simulink model "Dyn_6DoF_v2_0_R2015B"  (R2015b)
settings: Solver=ode4  SolverMode=SingleTasking  StartTime=0.0  StopTime=simInit.TSIM  FixedStep=simInit.dt  MaxStep=simInit.dt  RelTol=1e-3
InitFcn:
  | close all
undefined symbols (not defined in the file): act, base_windspeed, constr, DE2019, DiscIntNeverNeededParam, ENVMT, Lbooth, loiterStates, omega_rate_max, params, simInit, T, winchParameter
libraries: simulink x41, simulink_extras x4, dspsigops x1
(part 2 of 6)

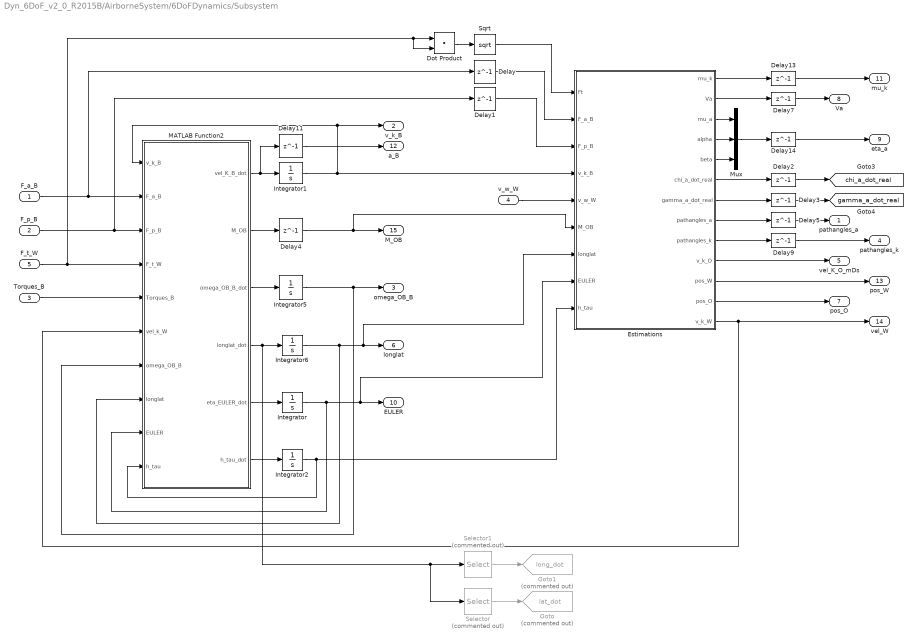
== system Dyn_6DoF_v2_0_R2015B/AirborneSystem/6DoFDynamics/Subsystem ==
  F_a_B : Inport  PortDimensions=[3,1]
  F_p_B : Inport  Port=2
  Torques_B : Inport  Port=3  PortDimensions=[3,1]
  v_w_W : Inport  Port=4  PortDimensions=[3,1]
  F_t_W : Inport  Port=5
  Delay{,1,11,14} (4 alike) : Delay  DelayLength=1  InitialCondition=zeros(3,1)
  Delay13 : Delay  DelayLength=1  InitialCondition=0
  Delay2 : Delay  DelayLength=1
  Delay3 : Delay  DelayLength=1
  Delay4 : Delay  DelayLength=1  InitialCondition=eye(3)
  Delay5 : Delay  DelayLength=1  InitialCondition=zeros(2,1)
  Delay7 : Delay  DelayLength=1  InitialCondition=simInit.vel_B_init(1)
  Delay9 : Delay  DelayLength=1  InitialCondition=zeros(2,1)
  Dot Product : DotProduct  InputSameDT=on  OutDataTypeStr=Inherit: Inherit via internal rule
  Estimations : MATLAB Function  TreatAsAtomicUnit=on
  Goto : Goto  Commented=on  GotoTag=lat_dot  TagVisibility=global
  Goto1 : Goto  Commented=on  GotoTag=long_dot  TagVisibility=global
  Integrator : Integrator  InitialCondition=simInit.eta_init  WrapState=on
  Integrator1 : Integrator  InitialCondition=simInit.vel_B_init
  Integrator2 : Integrator  InitialCondition=norm(simInit.pos_O_init)
  Integrator5 : Integrator  InitialCondition=zeros(3,1)
  Integrator6 : Integrator  InitialCondition=[simInit.long_init;simInit.lat_init]  WrapState=on
  MATLAB Function2 : MATLAB Function  TreatAsAtomicUnit=on
  Mux : Mux  Inputs=3
  Selector : Selector  Commented=on  InputPortWidth=2  IndexOptions=Index vector (dialog)  Indices=2  OutputSizes=1
  Selector1 : Selector  Commented=on  InputPortWidth=2  IndexOptions=Index vector (dialog)  Indices=1  OutputSizes=1
  Sqrt : Sqrt  SaturateOnIntegerOverflow=on
  pathangles_a : Outport  PortDimensions=[2,1]
  v_k_B : Outport  Port=2  PortDimensions=[3,1]
  omega_OB_B : Outport  Port=3  PortDimensions=[3,1]
  pathangles_k : Outport  Port=4  PortDimensions=[2,1]
  vel_K_O_mDs : Outport  Port=5  PortDimensions=[3,1]
  longlat : Outport  Port=6  PortDimensions=[2,1]
  pos_O : Outport  Port=7  PortDimensions=[3,1]
  Va : Outport  Port=8  PortDimensions=1
  eta_a : Outport  Port=9  PortDimensions=[3,1]
  EULER : Outport  Port=10  PortDimensions=[3,1]
  mu_k : Outport  Port=11  PortDimensions=1
  a_B : Outport  Port=12  PortDimensions=[3,1]
  pos_W : Outport  Port=13  PortDimensions=[3,1]
  vel_W : Outport  Port=14  PortDimensions=[3,1]
  M_OB : Outport  Port=15  PortDimensions=[3,3]
  tag scope: chi_a_dot_real=global, gamma_a_dot_real=global
  wires:
  Delay5/1 -> pathangles_a/1
  Delay4/1 -> M_OB/1, Estimations/6(M_OB)
  Torques_B/1 -> MATLAB Function2/5(Torques_B)
  MATLAB Function2/2(M_OB) -> Delay4/1
  F_a_B/1 -> MATLAB Function2/2(F_a_B), Delay/1
  Mux/1 -> Delay14/1
  MATLAB Function2/3(omega_OB_B_dot) -> Integrator5/1
  MATLAB Function2/4(longlat_dot) -> Integrator6/1, Selector/1, Selector1/1
  MATLAB Function2/1(vel_K_B_dot) -> Delay11/1, Integrator1/1
  v_w_W/1 -> Estimations/5(v_w_W)
  Integrator1/1 -> Estimations/4(v_k_B), MATLAB Function2/1(v_k_B), v_k_B/1
  F_p_B/1 -> MATLAB Function2/3(F_p_B), Delay1/1
  Estimations/8(pathangles_a) -> Delay5/1
  Estimations/9(pathangles_k) -> Delay9/1
  Estimations/2(Va) -> Delay7/1
  Delay7/1 -> Va/1
  Estimations/3(mu_a) -> Mux/1
  Delay2/1 -> [chi_a_dot_real]
  Estimations/6(chi_a_dot_real) -> Delay2/1
  Estimations/7(gamma_a_dot_real) -> Delay3/1
  Delay3/1 -> [gamma_a_dot_real]
  MATLAB Function2/5(eta_EULER_dot) -> Integrator/1
  Integrator/1 -> MATLAB Function2/9(EULER), Estimations/8(EULER), EULER/1
  Integrator5/1 -> MATLAB Function2/7(omega_OB_B), omega_OB_B/1
  Estimations/1(mu_k) -> Delay13/1
  Integrator6/1 -> MATLAB Function2/8(longlat), Estimations/7(longlat), longlat/1
  Delay13/1 -> mu_k/1
  Delay14/1 -> eta_a/1
  Delay9/1 -> pathangles_k/1
  Estimations/4(alpha) -> Mux/2
  Estimations/5(beta) -> Mux/3
  F_t_W/1 -> MATLAB Function2/4(F_t_W), Dot Product/1, Dot Product/2
  Dot Product/1 -> Sqrt/1
  Delay11/1 -> a_B/1
  MATLAB Function2/6(h_tau_dot) -> Integrator2/1
  Integrator2/1 -> MATLAB Function2/10(h_tau), Estimations/9(h_tau)
  Estimations/12(pos_O) -> pos_O/1
  Estimations/13(v_k_W) -> MATLAB Function2/6(vel_k_W), vel_W/1
  Estimations/11(pos_W) -> pos_W/1
  Estimations/10(v_k_O) -> vel_K_O_mDs/1
  Delay/1 -> Estimations/2(F_a_B)
  Delay1/1 -> Estimations/3(F_p_B)
  Sqrt/1 -> Estimations/1(Ft)
  Selector/1 -> Goto/1
  Selector1/1 -> Goto1/1

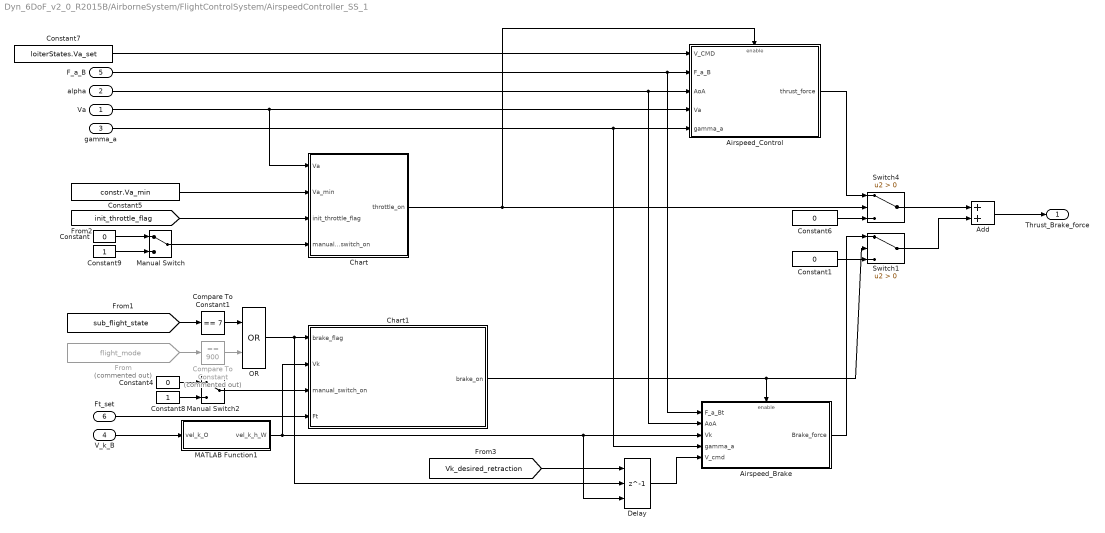
== system Dyn_6DoF_v2_0_R2015B/AirborneSystem/FlightControlSystem/AirspeedController_SS_1 ==
  Va : Inport
  alpha : Inport  Port=2
  gamma_a : Inport  Port=3
  V_k_B : Inport  Port=4
  F_a_B : Inport  Port=5
  Ft_set : Inport  Port=6
  Add : Sum
  Airspeed_Brake : Subsystem
  Airspeed_Control : Subsystem
  Chart : Stateflow chart  TreatAsAtomicUnit=on
  Chart1 : Stateflow chart  TreatAsAtomicUnit=on  mask{Ft_retract=params.F_t_retraction_set*params.F_t_traction_set, Vk_min=30}
      mask prompts: Ft_retract "Retraction force"; Vk_min "Minimum Vk"
  Compare To Constant : simulink/Logic and Bit Operations/Compare To Constant  Commented=on  relop===  const=900  OutDataTypeStr=boolean
  Compare To Constant1 : simulink/Logic and Bit Operations/Compare To Constant  relop===  const=7  OutDataTypeStr=boolean
  Constant{,1,4,6} (4 alike) : Constant  Value=0
  Constant5 : Constant  Value=constr.Va_min
  Constant7 : Constant  Value=loiterStates.Va_set
  Constant8 : Constant
  Constant9 : Constant
  Delay : Delay  DelayLength=1  InitialConditionSource=Input port  ExternalReset=Rising
      settings: InputPortMap=u0,r5,p4
  From : From  Commented=on  GotoTag=flight_mode  TagVisibility=global
  MATLAB Function1 : MATLAB Function  TreatAsAtomicUnit=on
  Manual Switch : ManualSwitch
  Manual Switch2 : ManualSwitch
  OR : Logic  Operator=OR  IconShape=distinctive  AllPortsSameDT=off  OutDataTypeStr=boolean
  Switch1 : Switch  Criteria=u2 > Threshold
  Switch4 : Switch  Criteria=u2 > Threshold
  Thrust_Brake_force : Outport
  wires:
  Switch1/1 -> Add/2
  Constant1/1 -> Switch1/3
  [Vk_desired_retraction] -> Delay/1
  Compare To Constant/1 -> OR/2
  Compare To Constant1/1 -> OR/1
  MATLAB Function1/1(vel_k_h_W) -> Chart1/2(Vk), Delay/3, Airspeed_Brake/3(Vk)
  V_k_B/1 -> MATLAB Function1/1(vel_k_O)
  Delay/1 -> Airspeed_Brake/5(V_cmd)
  Constant8/1 -> Manual Switch2/2
  Constant4/1 -> Manual Switch2/1
  Add/1 -> Thrust_Brake_force/1
  From/1 -> Compare To Constant/1
  [sub_flight_state] -> Compare To Constant1/1
  OR/1 -> Chart1/1(brake_flag), Delay/2
  Manual Switch2/1 -> Chart1/3(manual_switch_on)
  Ft_set/1 -> Chart1/4(Ft)
  Airspeed_Brake/1(Brake_force) -> Switch1/1
  Chart1/1(brake_on) -> Switch1/2, Airspeed_Brake/Enable
  Airspeed_Control/1(thrust_force) -> Switch4/1
  Constant5/1 -> Chart/2(Va_min)
  Va/1 -> Chart/1(Va), Airspeed_Control/4(Va)
  Chart/1(throttle_on) -> Switch4/2, Airspeed_Control/Enable
  Constant9/1 -> Manual Switch/2
  [init_throttle_flag] -> Chart/3(init_throttle_flag)
  alpha/1 -> Airspeed_Control/3(AoA), Airspeed_Brake/2(AoA)
  Constant7/1 -> Airspeed_Control/1(V_CMD)
  Manual Switch/1 -> Chart/4(manual_switch_on)
  Constant/1 -> Manual Switch/1
  Constant6/1 -> Switch4/3
  F_a_B/1 -> Airspeed_Control/2(F_a_B), Airspeed_Brake/1(F_a_Bt)
  gamma_a/1 -> Airspeed_Control/5(gamma_a), Airspeed_Brake/4(gamma_a)
  Switch4/1 -> Add/1

== system Dyn_6DoF_v2_0_R2015B/AirborneSystem/FlightControlSystem/AttitudeAndRateLoop ==
  mu_a_cmd : Inport
  M_a_B_est : Inport  Port=2
  flightMode : Inport  Port=3
  alpha_a_cmd : Inport  Port=4
  StateEstimation_Bus : Inport  Port=5
  AttitudeController : Subsystem
  Compare To Constant : simulink/Logic and Bit Operations/Compare To Constant  relop===  const=6  OutDataTypeStr=boolean
  RateLoop : Subsystem
  u_rb : Outport
  wires:
  M_a_B_est/1 -> RateLoop/3(M_a_B_est)
  RateLoop/1(u_rb) -> u_rb/1
  mu_a_cmd/1 -> AttitudeController/2(mu_a_cmd)
  AttitudeController/1(omega_OB_B_cmd) -> RateLoop/2(omega_OB_B_cmd)
  alpha_a_cmd/1 -> AttitudeController/3(alpha_a_cmd)
  StateEstimation_Bus/1 -> RateLoop/1(StateEstimation_Bus), AttitudeController/1(StateEstimation_Bus)
  flightMode/1 -> Compare To Constant/1
  Compare To Constant/1 -> AttitudeController/4(reset)

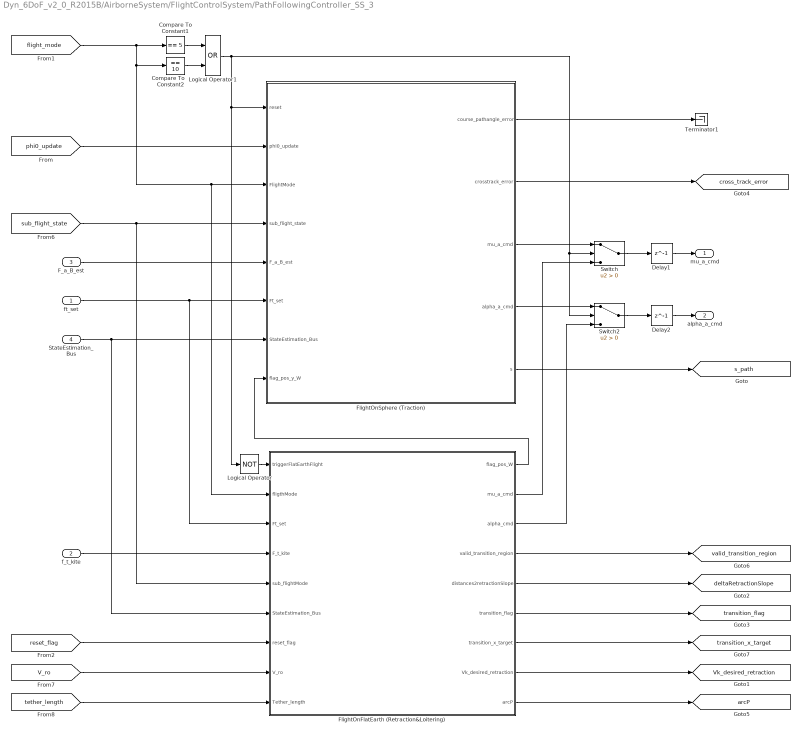
== system Dyn_6DoF_v2_0_R2015B/AirborneSystem/FlightControlSystem/PathFollowingController_SS_3 ==
  ft_set : Inport
  f_t_kite : Inport  Port=2
  F_a_B_est : Inport  Port=3  PortDimensions=[3,1]
  StateEstimation_Bus : Inport  Port=4
  Compare To Constant1 : simulink/Logic and Bit Operations/Compare To Constant  relop===  const=5  OutDataTypeStr=boolean
  Compare To Constant2 : simulink/Logic and Bit Operations/Compare To Constant  relop===  const=10  OutDataTypeStr=boolean
  Delay1 : Delay  DelayLength=1
  Delay2 : Delay  DelayLength=1
  FlightOnFlatEarth (Retraction&Loitering) : Subsystem
  FlightOnSphere (Traction) : Subsystem
  Logical Operator : Logic  Operator=NOT  AllPortsSameDT=off  OutDataTypeStr=boolean
  Logical Operator1 : Logic  Operator=OR  AllPortsSameDT=off  OutDataTypeStr=boolean
  Switch : Switch  Criteria=u2 > Threshold
  Switch2 : Switch  Criteria=u2 > Threshold
  Terminator1 : Terminator
  mu_a_cmd : Outport  PortDimensions=1
  alpha_a_cmd : Outport  Port=2  PortDimensions=1
  tag scope: Vk_desired_retraction=global, arcP=global, cross_track_error=global, deltaRetractionSlope=global, s_path=global, transition_flag=global, transition_x_target=global, valid_transition_region=global
  wires:
  FlightOnFlatEarth (Retraction&Loitering)/9(arcP) -> [arcP]
  [sub_flight_state] -> FlightOnSphere (Traction)/4(sub_flight_state), FlightOnFlatEarth (Retraction&Loitering)/5(sub_flightMode)
  [tether_length] -> FlightOnFlatEarth (Retraction&Loitering)/9(Tether_length)
  [V_ro] -> FlightOnFlatEarth (Retraction&Loitering)/8(V_ro)
  FlightOnFlatEarth (Retraction&Loitering)/8(Vk_desired_retraction) -> [Vk_desired_retraction]
  FlightOnFlatEarth (Retraction&Loitering)/7(transition_x_target) -> [transition_x_target]
  FlightOnFlatEarth (Retraction&Loitering)/1(flag_pos_W) -> FlightOnSphere (Traction)/8(flag_pos_y_W)
  FlightOnFlatEarth (Retraction&Loitering)/5(distances2retractionSlope) -> [deltaRetractionSlope]
  [reset_flag] -> FlightOnFlatEarth (Retraction&Loitering)/7(reset_flag)
  FlightOnFlatEarth (Retraction&Loitering)/6(transition_flag) -> [transition_flag]
  [phi0_update] -> FlightOnSphere (Traction)/2(phi0_update)
  FlightOnSphere (Traction)/5(s) -> [s_path]
  Compare To Constant2/1 -> Logical Operator1/2
  Compare To Constant1/1 -> Logical Operator1/1
  [flight_mode] -> Compare To Constant2/1, FlightOnSphere (Traction)/3(FlightMode), FlightOnFlatEarth (Retraction&Loitering)/2(fligthMode), Compare To Constant1/1
  FlightOnSphere (Traction)/2(crosstrack_error) -> [cross_track_error]
  FlightOnSphere (Traction)/1(course_pathangle_error) -> Terminator1/1
  FlightOnSphere (Traction)/3(mu_a_cmd) -> Switch/1
  FlightOnSphere (Traction)/4(alpha_a_cmd) -> Switch2/1
  F_a_B_est/1 -> FlightOnSphere (Traction)/5(F_a_B_est)
  f_t_kite/1 -> FlightOnFlatEarth (Retraction&Loitering)/4(F_t_kite)
  Switch2/1 -> Delay2/1
  Switch/1 -> Delay1/1
  Delay1/1 -> mu_a_cmd/1
  Delay2/1 -> alpha_a_cmd/1
  ft_set/1 -> FlightOnSphere (Traction)/6(Ft_set), FlightOnFlatEarth (Retraction&Loitering)/3(Ft_set)
  Logical Operator/1 -> FlightOnFlatEarth (Retraction&Loitering)/1(triggerFlatEarthFlight)
  FlightOnFlatEarth (Retraction&Loitering)/2(mu_a_cmd) -> Switch/3
  FlightOnFlatEarth (Retraction&Loitering)/3(alpha_cmd) -> Switch2/3
  FlightOnFlatEarth (Retraction&Loitering)/4(valid_transition_region) -> [valid_transition_region]
  Logical Operator1/1 -> Switch2/2, Switch/2, Logical Operator/1, FlightOnSphere (Traction)/1(reset)
  StateEstimation_Bus/1 -> FlightOnFlatEarth (Retraction&Loitering)/6(StateEstimation_Bus), FlightOnSphere (Traction)/7(StateEstimation_Bus)

== system Dyn_6DoF_v2_0_R2015B/AirborneSystem/ForcesAndTorques/Subsystem Reference_SS_4 ==
  u_cmd : Inport
  Aileron1 : Subsystem  mask(Rate and Position Limited Servo){freq=act.aileron.w0/(2*pi), RL=act.aileron.rl, POS_hi=act.aileron.max_deflection, POS_lo=act.aileron.min_deflection, Bias=act.aileron.bias}
      mask prompts: freq "Bandwidth, Hz"; RL "Rate Limit:"; POS_hi "Position Limit High:"; POS_lo "Position Limit Low:"; Bias "Bias Value:"
      mask help:
      | First order transfer function: w/(s+w), with rate and position limits
      | and output bias level.
      mask Display:
      | text(.48,.55,sprintf('%3.1f Hz\nBW',freq),'horizontalAlignment','center');
      | 
      | text(0.18,0.45,sprintf('|d/dt|\n<%0.1f',RL),'horizontalAlignment','center');
      | 
      | text(0.88,0.85,num2str(POS_hi),'horizontalAlignment', 'center');
      | text(0.88,0.2,num2str(POS_lo),'horizontalAlignment', 'center');
      | text(0.73,0.5,'P\nL');
      | 
      | 
      | plot([0.83 0.87 0.93 0.97],[0.4 0.4 0.6 0.6]);
      | plot([0.81 0.99],[0.5 0.5]);
      | plot([0.9 0.9],[0.3 0.7]);
      | plot([0.81 0.99 0.99 0.81 0.81],[0.3 0.3 0.7 0.7 0.3]);
  Delay1 : Delay  Commented=on  DelayLength=1  InitialCondition=0
  Delay2 : Delay  Commented=on  DelayLength=1  InitialCondition=0
  Delay3 : Delay  Commented=on  DelayLength=1  InitialCondition=0
  Delay4 : Delay  DelayLength=1  InitialCondition=0
  Delay5 : Delay  DelayLength=1  InitialCondition=0
  Delay6 : Delay  DelayLength=1  InitialCondition=0
  Demux : Demux  Outputs=3
  Elevator : Subsystem  mask(Rate and Position Limited Servo){freq=act.elevator.w0/(2*pi), RL=act.elevator.rl, POS_hi=act.elevator.max_deflection, POS_lo=act.elevator.min_deflection, Bias=act.elevator.bias}
      mask prompts: freq "Bandwidth, Hz"; RL "Rate Limit:"; POS_hi "Position Limit High:"; POS_lo "Position Limit Low:"; Bias "Bias Value:"
      mask help:
      | First order transfer function: w/(s+w), with rate and position limits
      | and output bias level.
      mask Display:
      | text(.48,.55,sprintf('%3.1f Hz\nBW',freq),'horizontalAlignment','center');
      | 
      | text(0.18,0.45,sprintf('|d/dt|\n<%0.1f',RL),'horizontalAlignment','center');
      | 
      | text(0.88,0.85,num2str(POS_hi),'horizontalAlignment', 'center');
      | text(0.88,0.2,num2str(POS_lo),'horizontalAlignment', 'center');
      | text(0.73,0.5,'P\nL');
      | 
      | 
      | plot([0.83 0.87 0.93 0.97],[0.4 0.4 0.6 0.6]);
      | plot([0.81 0.99],[0.5 0.5]);
      | plot([0.9 0.9],[0.3 0.7]);
      | plot([0.81 0.99 0.99 0.81 0.81],[0.3 0.3 0.7 0.7 0.3]);
  Manual Switch : ManualSwitch  CurrentSetting=0
  Mux1 : Mux  Inputs=3
  Mux2 : Mux  Inputs=3
  Rudder1 : Subsystem  mask(Rate and Position Limited Servo){freq=act.rudder.w0/(2*pi), RL=act.rudder.rl, POS_hi=act.rudder.max_deflection, POS_lo=act.rudder.min_deflection, Bias=act.rudder.bias}
      mask prompts: freq "Bandwidth, Hz"; RL "Rate Limit:"; POS_hi "Position Limit High:"; POS_lo "Position Limit Low:"; Bias "Bias Value:"
      mask help:
      | First order transfer function: w/(s+w), with rate and position limits
      | and output bias level.
      mask Display:
      | text(.48,.55,sprintf('%3.1f Hz\nBW',freq),'horizontalAlignment','center');
      | 
      | text(0.18,0.45,sprintf('|d/dt|\n<%0.1f',RL),'horizontalAlignment','center');
      | 
      | text(0.88,0.85,num2str(POS_hi),'horizontalAlignment', 'center');
      | text(0.88,0.2,num2str(POS_lo),'horizontalAlignment', 'center');
      | text(0.73,0.5,'P\nL');
      | 
      | 
      | plot([0.83 0.87 0.93 0.97],[0.4 0.4 0.6 0.6]);
      | plot([0.81 0.99],[0.5 0.5]);
      | plot([0.9 0.9],[0.3 0.7]);
      | plot([0.81 0.99 0.99 0.81 0.81],[0.3 0.3 0.7 0.7 0.3]);
  Saturation : Saturate  Commented=on  UpperLimit=act.aileron.max_deflection  LowerLimit=act.aileron.min_deflection
  Saturation1 : Saturate  Commented=on  UpperLimit=act.elevator.max_deflection  LowerLimit=act.elevator.min_deflection
  Saturation2 : Saturate  Commented=on  UpperLimit=act.rudder.max_deflection  LowerLimit=act.rudder.min_deflection
  Saturation4 : Saturate  UpperLimit=act.elevator.max_deflection  LowerLimit=act.elevator.min_deflection
  Saturation6 : Saturate  UpperLimit=act.aileron.max_deflection  LowerLimit=act.aileron.min_deflection
  Saturation7 : Saturate  UpperLimit=act.rudder.max_deflection  LowerLimit=act.rudder.min_deflection
  Act_out_est : Outport
  wires:
  Delay3/1 -> Saturation2/1
  Mux2/1 -> Manual Switch/2
  Saturation1/1 -> Mux1/2
  Delay4/1 -> Saturation6/1
  Delay1/1 -> Saturation/1
  Manual Switch/1 -> Act_out_est/1
  Saturation6/1 -> Aileron1/1(In)
  Saturation/1 -> Mux1/1
  Saturation7/1 -> Rudder1/1(In)
  Rudder1/1(Out) -> Mux2/3
  Elevator/1(Out) -> Mux2/2
  Delay5/1 -> Saturation4/1
  Demux/2 -> Delay5/1, Delay2/1
  Mux1/1 -> Manual Switch/1
  Demux/1 -> Delay1/1, Delay4/1
  Delay6/1 -> Saturation7/1
  Delay2/1 -> Saturation1/1
  Saturation4/1 -> Elevator/1(In)
  Saturation2/1 -> Mux1/3
  u_cmd/1 -> Demux/1
  Aileron1/1(Out) -> Mux2/1
  Demux/3 -> Delay6/1, Delay3/1

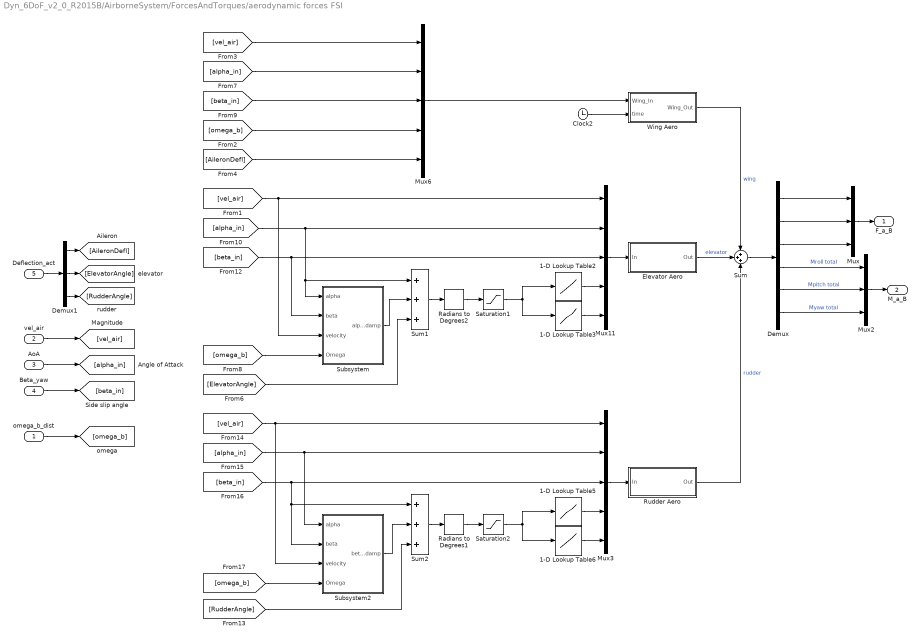
== system Dyn_6DoF_v2_0_R2015B/AirborneSystem/ForcesAndTorques/aerodynamic forces FSI ==
  omega_b_dist : Inport
  vel_air : Inport  Port=2
  AoA : Inport  Port=3
  Beta_yaw : Inport  Port=4
  Deflection_act : Inport  Port=5
  1-D Lookup Table2 : Lookup_n-D  NumberOfTableDimensions=1  BreakpointsForDimension1=DE2019.alpha  BreakpointsForDimension2=[1 1]  Table=DE2019.el_cL'  InternalRulePriority=Speed  RndMeth=Simplest  InputSameDT=on
  1-D Lookup Table3 : Lookup_n-D  NumberOfTableDimensions=1  BreakpointsForDimension1=DE2019.alpha  BreakpointsForDimension2=[1 1]  Table=DE2019.el_cD'  InternalRulePriority=Speed  RndMeth=Simplest  InputSameDT=on
  1-D Lookup Table5 : Lookup_n-D  NumberOfTableDimensions=1  BreakpointsForDimension1=DE2019.alpha  BreakpointsForDimension2=[1 1]  Table=DE2019.vs_cL'  InternalRulePriority=Speed  RndMeth=Simplest  InputSameDT=on
  1-D Lookup Table6 : Lookup_n-D  NumberOfTableDimensions=1  BreakpointsForDimension1=DE2019.alpha  BreakpointsForDimension2=[1 1]  Table=DE2019.vs_cD'  InternalRulePriority=Speed  RndMeth=Simplest  InputSameDT=on
  Clock2 : Clock
  Demux : Demux  Outputs=6
  Demux1 : Demux  Outputs=3
  Elevator Aero : Subsystem
  Mux : Mux  Inputs=3
  Mux11 : Mux  Inputs=5
  Mux2 : Mux  Inputs=3
  Mux3 : Mux  Inputs=5
  Mux6 : Mux  Inputs=5
  Radians to Degrees1 : simulink_extras/Transformations/Radians to Degrees
  Radians to Degrees2 : simulink_extras/Transformations/Radians to Degrees
  Rudder Aero : Subsystem
  Saturation1 : Saturate  UpperLimit=max(DE2019.alpha)  LowerLimit=min(DE2019.alpha)
  Saturation2 : Saturate  UpperLimit=max(DE2019.alpha)  LowerLimit=min(DE2019.alpha)
  Subsystem : Subsystem
  Subsystem2 : Subsystem
  Sum : Sum  Inputs=+++
  Sum1 : Sum  Inputs=+++
  Sum2 : Sum  Inputs=+++
  Wing Aero : Subsystem  TreatAsAtomicUnit=on  SystemSampleTime=0.01
  F_a_B : Outport
  M_a_B : Outport  Port=2
  wires:
  Sum/1 -> Demux/1
  Mux6/1 -> Wing Aero/1(Wing_In)
  omega_b_dist/1 -> [omega_b]
  Demux1/2 -> [ElevatorAngle]
  vel_air/1 -> [vel_air]
  [vel_air] -> Subsystem/3(velocity), Mux11/1
  Clock2/1 -> Wing Aero/2(time)
  Elevator Aero/1(Out) -> Sum/2  "elevator"
  Wing Aero/1(Wing_Out) -> Sum/1  "wing"
  Deflection_act/1 -> Demux1/1
  Demux1/1 -> [AileronDefl]
  Demux1/3 -> [RudderAngle]
  AoA/1 -> [alpha_in]
  Beta_yaw/1 -> [beta_in]
  [ElevatorAngle] -> Sum1/3
  [omega_b] -> Subsystem/4(Omega)
  [alpha_in] -> Subsystem/1(alpha), Sum1/1, Mux11/2
  [beta_in] -> Subsystem/2(beta), Mux11/3
  Demux/1 -> Mux/1
  Demux/2 -> Mux/2
  Demux/3 -> Mux/3
  Mux/1 -> F_a_B/1
  Demux/6 -> Mux2/3  "Myaw total"
  Mux2/1 -> M_a_B/1
  Demux/4 -> Mux2/1  "Mroll total"
  Demux/5 -> Mux2/2  "Mpitch total"
  Sum1/1 -> Radians to Degrees2/1
  Radians to Degrees2/1 -> Saturation1/1
  Saturation1/1 -> 1-D Lookup Table2/1, 1-D Lookup Table3/1
  Subsystem/1(alpha_damp) -> Sum1/2
  1-D Lookup Table2/1 -> Mux11/4
  1-D Lookup Table3/1 -> Mux11/5
  Mux11/1 -> Elevator Aero/1(In)
  Radians to Degrees1/1 -> Saturation2/1
  [alpha_in] -> Subsystem2/1(alpha), Mux3/2
  [beta_in] -> Subsystem2/2(beta), Sum2/1, Mux3/3
  [RudderAngle] -> Sum2/3
  [omega_b] -> Subsystem2/4(Omega)
  Saturation2/1 -> 1-D Lookup Table6/1, 1-D Lookup Table5/1
  [vel_air] -> Subsystem2/3(velocity), Mux3/1
  Subsystem2/1(beta_damp) -> Sum2/2
  1-D Lookup Table6/1 -> Mux3/5
  1-D Lookup Table5/1 -> Mux3/4
  Sum2/1 -> Radians to Degrees1/1
  Mux3/1 -> Rudder Aero/1(In)
  Rudder Aero/1(Out) -> Sum/3  "rudder"
  [vel_air] -> Mux6/1
  [alpha_in] -> Mux6/2
  [beta_in] -> Mux6/3
  [omega_b] -> Mux6/4
  [AileronDefl] -> Mux6/5

== system Dyn_6DoF_v2_0_R2015B/Environment_SS_5/Windshear/Wind Shear Model ==
  Altitude : Inport
  DCM : Inport  Port=2  PortDimensions=[3 3]
  Degrees to Radians : simulink_extras/Transformations/Degrees to Radians
  Disallow CGS : UnitConfiguration  UnitSystemsStr=English,SI,SI (extended)  AllowAllUnitSystems=off
  Mux : Mux  Inputs=3
  Reshape1 : Reshape
  SinCos : Trigonometry  Operator=sincos
  Transform from Inertial to Body axes : Product  Inputs=**  Multiplication=Matrix(*)  SaturateOnIntegerOverflow=on  InputSameDT=on  OutDataTypeStr=Inherit: Same as first input
  Wdeg1 : Constant  Value=0  OutDataTypeStr=Inherit: Inherit via back propagation
  Wind Direction : Constant  Value=ENVMT.windDirection_rad*180/pi  OutDataTypeStr=Inherit: Inherit via back propagation
  Wind speed at reference height : Gain  Gain=-base_windspeed  SaturateOnIntegerOverflow=on  OutDataTypeStr=Inherit: Same as input  ParamDataTypeStr=Inherit: Same as input
  wind_field_calc : Subsystem
  Mean Wind : Outport
  wires:
  Reshape1/1 -> Mean Wind/1
  wind_field_calc/1(Windspeed_altitude) -> Transform from Inertial to Body axes/2
  Degrees to Radians/1 -> SinCos/1
  Wind speed at reference height/1 -> wind_field_calc/2(Base_windspeed)
  DCM/1 -> Transform from Inertial to Body axes/1
  Mux/1 -> Wind speed at reference height/1
  Wdeg1/1 -> Mux/3  "Wz"
  SinCos/1 -> Mux/2  "Wy"
  SinCos/2 -> Mux/1  "Wx"
  Wind Direction/1 -> Degrees to Radians/1
  Transform from Inertial to Body axes/1 -> Reshape1/1
  Altitude/1 -> wind_field_calc/1(Altitude)

== system Dyn_6DoF_v2_0_R2015B/Environment_SS_5/wind_field_calc/Length Conversion ==
  in : Inport
  Unit Conversion : UnitConversion
  out : Outport
  wires:
  Unit Conversion/1 -> out/1
  in/1 -> Unit Conversion/1

== system Dyn_6DoF_v2_0_R2015B/Subsystem WinchControl_SS_8/PureTorqueControl/PI-ForceController ==
  RetractionFlag : Inport
  controlDeficitDue2Sat : Inport  Port=2
  e_Ft : Inport  Port=3
  Abs : Abs
  Compare To Constant : simulink/Logic and Bit Operations/Compare To Constant  relop=>=  const=1e-3  OutDataTypeStr=boolean
  Constant2 : Constant  Value=0
  Gain8 : Gain  Gain=params.ki_winch
  Gain9 : Gain  Gain=params.kp_winch
  Integrator : Integrator
  Logical Operator : Logic  Operator=OR  AllPortsSameDT=off  OutDataTypeStr=boolean
  Sum8 : Sum
  Switch : Switch  Criteria=u2 > Threshold
  TorqueCmd : Outport
  wires:
  Sum8/1 -> TorqueCmd/1
  Switch/1 -> Integrator/1
  Constant2/1 -> Switch/1
  Gain9/1 -> Sum8/2
  Gain8/1 -> Switch/3
  Compare To Constant/1 -> Logical Operator/2
  Integrator/1 -> Sum8/1
  Abs/1 -> Compare To Constant/1
  e_Ft/1 -> Gain8/1, Gain9/1
  controlDeficitDue2Sat/1 -> Abs/1
  RetractionFlag/1 -> Logical Operator/1
  Logical Operator/1 -> Switch/2

== system Dyn_6DoF_v2_0_R2015B/AirborneSystem/FlightControlSystem/AirspeedController_SS_1/Airspeed_Brake ==
  F_a_Bt : Inport  PortDimensions=[3,1]
  AoA : Inport  Port=2
  Vk : Inport  Port=3
  gamma_a : Inport  Port=4
  V_cmd : Inport  Port=5
  Enable : EnablePort
  Delay1 : Delay  DelayLength=1  InitialConditionSource=Input port  InitialCondition=zeros(3,1)
      settings: InputPortMap=u0,p4
  Discrete-Time Integrator : DiscreteIntegrator  InitialConditionSetting=State (most efficient)  SampleTime=-1  ICPrevOutput=DiscIntNeverNeededParam  ICPrevScaledInput=DiscIntNeverNeededParam
  FeedforwardPart : MATLAB Function  TreatAsAtomicUnit=on
  Gain3 : Gain  Gain=params.Kp_brake
  Gain4 : Gain  Gain=params.Ki_brake
  MATLAB Function : MATLAB Function  TreatAsAtomicUnit=on
  Saturation : Saturate  UpperLimit=0  LowerLimit=-inf  LinearizeAsGain=off
  Scope : Scope  NumInputPorts=3
  Scope1 : Scope
  Subsystem : Subsystem
  Sum1 : Sum
  Sum2 : Sum  Inputs=|+-
  Sum3 : Sum  Inputs=-+|
  hedging : MATLAB Function  TreatAsAtomicUnit=on
  Brake_force : Outport
  wires:
  AoA/1 -> MATLAB Function/2(AoA)
  MATLAB Function/1(Drag) -> FeedforwardPart/3(Drag_force), hedging/1(Drag_force)
  F_a_Bt/1 -> MATLAB Function/1(F_a_B)
  Sum2/1 -> Subsystem/2(v_h)
  hedging/1(nu_V) -> Sum2/2
  FeedforwardPart/1(BF) -> Saturation/1
  Saturation/1 -> Brake_force/1, Scope1/1, hedging/3(BF)
  Sum1/1 -> Sum2/1, FeedforwardPart/2(nu_V)
  Subsystem/1(V_k_ref) -> Scope/3, Sum3/2
  gamma_a/1 -> hedging/2(gamma), FeedforwardPart/1(gamma)
  Sum3/1 -> Gain4/1, Gain3/1
  Gain3/1 -> Sum1/1
  Discrete-Time Integrator/1 -> Sum1/2
  Gain4/1 -> Discrete-Time Integrator/1
  V_cmd/1 -> Scope/1, Subsystem/1(V_cmd)
  Delay1/1 -> Subsystem/3(Initial), Delay1/1
  Vk/1 -> Delay1/2, Sum3/1, Scope/2

== system Dyn_6DoF_v2_0_R2015B/AirborneSystem/FlightControlSystem/AirspeedController_SS_1/Airspeed_Control ==
  V_CMD : Inport
  F_a_B : Inport  Port=2  PortDimensions=[3,1]
  AoA : Inport  Port=3
  Va : Inport  Port=4
  gamma_a : Inport  Port=5
  Enable : EnablePort
  Discrete-Time Integrator : DiscreteIntegrator  InitialConditionSetting=State (most efficient)  SampleTime=-1  ICPrevOutput=DiscIntNeverNeededParam  ICPrevScaledInput=DiscIntNeverNeededParam
  FeedforwardPart : MATLAB Function  TreatAsAtomicUnit=on
  Gain3 : Gain  Gain=params.kp_speed_control
  Gain4 : Gain  Gain=params.ki_speed_control
  MATLAB Function : MATLAB Function  TreatAsAtomicUnit=on
  Saturation : Saturate  UpperLimit=inf  LowerLimit=0  LinearizeAsGain=off
  Scope : Scope  NumInputPorts=3
  Subsystem : Subsystem
  Sum : Sum  Inputs=-+|
  Sum1 : Sum  Inputs=+++
  Sum2 : Sum  Inputs=|+-
  hedging : MATLAB Function  TreatAsAtomicUnit=on
  thrust_force : Outport
  wires:
  AoA/1 -> MATLAB Function/2(AoA)
  MATLAB Function/1(Drag) -> hedging/1(Drag_force), FeedforwardPart/3(Drag_force)
  F_a_B/1 -> MATLAB Function/1(F_a_B)
  Sum2/1 -> Subsystem/2(v_h)
  hedging/1(nu_V) -> Sum2/2
  FeedforwardPart/1(T) -> Saturation/1
  Saturation/1 -> thrust_force/1, hedging/3(T)
  Subsystem/1(V_k_ref_dot) -> Sum1/1
  Sum1/1 -> Sum2/1, FeedforwardPart/2(nu_V)
  Subsystem/2(V_k_ref) -> Sum/2, Scope/3
  gamma_a/1 -> hedging/2(gamma), FeedforwardPart/1(gamma)
  V_CMD/1 -> Subsystem/1(V_cmd), Scope/1
  Sum/1 -> Gain4/1, Gain3/1
  Va/1 -> Scope/2, Sum/1
  Gain3/1 -> Sum1/2
  Discrete-Time Integrator/1 -> Sum1/3
  Gain4/1 -> Discrete-Time Integrator/1

== system Dyn_6DoF_v2_0_R2015B/AirborneSystem/FlightControlSystem/AttitudeAndRateLoop/AttitudeController ==
  StateEstimation_Bus : Inport
  mu_a_cmd : Inport  Port=2
  alpha_a_cmd : Inport  Port=3
  reset : Inport  Port=4
  Bus Selector : BusSelector  OutputSignals=airdata,mu_a,pathangles_a
  Demux : Demux  Outputs=3
  Gain1 : Gain  Commented=on  Gain=180/pi
  InversionAttitude : MATLAB Function  TreatAsAtomicUnit=on
  Mux : Mux  Inputs=3
  PI-controller : Subsystem  mask{Kp_mu=params.Kp_mu, Kp_alpha=params.Kp_alpha, Kp_beta=params.Kp_beta, Ki_mu=params.Ki_mu, Ki_alpha=params.Ki_alpha, Ki_beta=params.Ki_beta}
  Scope3 : Scope  Commented=on
  SecondOrderReferenceModel_alpha_a : Subsystem  mask{omega0_max=params.w0_alpha, zeta0=1, y_max=constr.alpha_a_max, y_min=constr.alpha_a_min, yd_max=inf, yd_min=-inf, y2d_max=inf, y2d_min=-inf}
  SecondOrderReferenceModel_mu_a : Subsystem  mask{omega0_max=params.w0_mu, zeta0=1, y_max=constr.mu_a_max, y_min=constr.mu_a_min, yd_max=inf, yd_min=-inf, y2d_max=inf, y2d_min=-inf}
  Selector : Selector  InputPortWidth=3  IndexOptions=Index vector (dialog)  Indices=2  OutputSizes=1
  Selector1 : Selector  InputPortWidth=3  IndexOptions=Index vector (dialog)  Indices=3  OutputSizes=1
  Selector2 : Selector  InputPortWidth=2  IndexOptions=Index vector (dialog)  Indices=2  OutputSizes=1
  Sum : Sum  Inputs=|+-
  Terminator : Terminator
  alpha_control : Scope  Commented=on  NumInputPorts=3
  mu_control : Scope  Commented=on  NumInputPorts=3
  omega_OB_B_cmd : Outport  PortDimensions=[3,1]
  wires:
  Demux/2 -> SecondOrderReferenceModel_alpha_a/2(hedge)
  Demux/1 -> SecondOrderReferenceModel_mu_a/2(hedge)
  Sum/1 -> Demux/1
  InversionAttitude/2(nu_hat) -> Sum/2
  Mux/1 -> Sum/1
  mu_a_cmd/1 -> mu_control/1, SecondOrderReferenceModel_mu_a/1(y_cmd)
  alpha_a_cmd/1 -> alpha_control/1, SecondOrderReferenceModel_alpha_a/1(y_cmd)
  Selector2/1 -> InversionAttitude/9(gamma_a)
  Bus Selector/3 -> Selector2/1  "<pathangles_a>"
  Bus Selector/2 -> mu_control/3, PI-controller/3(mu_a), InversionAttitude/1(mu_a)  "<mu_a>"
  Bus Selector/1 -> Selector/1, Selector1/1  "<airdata>"
  StateEstimation_Bus/1 -> Bus Selector/1
  [gamma_a_dot_real] -> InversionAttitude/8(gamma_a_dot_real)
  [chi_a_dot_real] -> InversionAttitude/7(chi_a_dot_real)
  InversionAttitude/1(omega_OB_B_cmd) -> omega_OB_B_cmd/1
  PI-controller/1(nu_beta) -> InversionAttitude/6(nu_beta_a), Mux/3
  PI-controller/3(nu_mu) -> InversionAttitude/4(nu_mu_a), Mux/1
  SecondOrderReferenceModel_mu_a/1(y_ref) -> PI-controller/1(mu_ref), mu_control/2
  SecondOrderReferenceModel_mu_a/2(y_ref_dot) -> PI-controller/2(mu_dot_ref)
  SecondOrderReferenceModel_alpha_a/1(y_ref) -> alpha_control/2, PI-controller/4(alpha_ref)
  SecondOrderReferenceModel_alpha_a/2(y_ref_dot) -> PI-controller/5(alpha_dot_ref)
  PI-controller/2(nu_alpha) -> InversionAttitude/5(nu_alpha_a), Mux/2
  reset/1 -> PI-controller/6(reset)
  Demux/3 -> Terminator/1
  Selector/1 -> InversionAttitude/2(alpha), PI-controller/7(alpha), alpha_control/3
  Selector1/1 -> InversionAttitude/3(beta), Gain1/1, PI-controller/8(beta)
  Gain1/1 -> Scope3/1

== system Dyn_6DoF_v2_0_R2015B/AirborneSystem/FlightControlSystem/AttitudeAndRateLoop/RateLoop ==
  StateEstimation_Bus : Inport
  omega_OB_B_cmd : Inport  Port=2
  M_a_B_est : Inport  Port=3
  Actuatormodel _SS_2 : Subsystem
  Bus Selector : BusSelector  OutputSignals=airdata,omega_OB_B
  ControlAllocation : Subsystem
  Rate_Loop : Subsystem
  u_rb : Outport
  wires:
  Bus Selector/2 -> Rate_Loop/1(omega_OB_B)  "<omega_OB_B>"
  omega_OB_B_cmd/1 -> Rate_Loop/2(omega_OB_B_cmd)
  StateEstimation_Bus/1 -> Bus Selector/1
  Rate_Loop/1(delta_M_cmd) -> ControlAllocation/3(Delta_mom_cmd)
  M_a_B_est/1 -> Rate_Loop/3(M_a_B_est)
  Bus Selector/1 -> ControlAllocation/2(airdata)  "<airdata>"
  Actuatormodel _SS_2/1(Act_out_est) -> ControlAllocation/1(deflections_actuator_output)
  ControlAllocation/1(deflections_cmd) -> u_rb/1, Actuatormodel _SS_2/1(u_cmd)

== system Dyn_6DoF_v2_0_R2015B/AirborneSystem/FlightControlSystem/PathFollowingController_SS_3/FlightOnFlatEarth (Retraction&Loitering) ==
  triggerFlatEarthFlight : Inport
  fligthMode : Inport  Port=2
  Ft_set : Inport  Port=3
  F_t_kite : Inport  Port=4
  sub_flightMode : Inport  Port=5
  StateEstimation_Bus : Inport  Port=6
  reset_flag : Inport  Port=7
  V_ro : Inport  Port=8
  Tether_length : Inport  Port=9
  CalculateAttitudeCmds : Subsystem
  GuidanceFlatEarth : Subsystem
  flag_pos_W : Outport
  mu_a_cmd : Outport  Port=2
  alpha_cmd : Outport  Port=3
  valid_transition_region : Outport  Port=4
  distances2retractionSlope : Outport  Port=5
  transition_flag : Outport  Port=6
  transition_x_target : Outport  Port=7
  Vk_desired_retraction : Outport  Port=8
  arcP : Outport  Port=9
  wires:
  StateEstimation_Bus/1 -> CalculateAttitudeCmds/7(StateEstimation_Bus), GuidanceFlatEarth/2(StateEstimation_Bus)
  CalculateAttitudeCmds/1(mu_a_cmd) -> mu_a_cmd/1
  Ft_set/1 -> CalculateAttitudeCmds/3(Ft_set)
  CalculateAttitudeCmds/2(alpha_cmd) -> alpha_cmd/1
  fligthMode/1 -> CalculateAttitudeCmds/6(flightMode), GuidanceFlatEarth/1(flightMode)
  triggerFlatEarthFlight/1 -> GuidanceFlatEarth/Enable, CalculateAttitudeCmds/1(flight_on_flatearth_flag)
  GuidanceFlatEarth/3(valid_transition_region) -> valid_transition_region/1
  F_t_kite/1 -> CalculateAttitudeCmds/4(F_t_kite)
  GuidanceFlatEarth/1(distances2slope) -> distances2retractionSlope/1
  GuidanceFlatEarth/2(course_path) -> CalculateAttitudeCmds/2(pathangles_k_cmd)
  sub_flightMode/1 -> CalculateAttitudeCmds/5(sub_flightMode)
  GuidanceFlatEarth/4(transition_flag) -> transition_flag/1
  reset_flag/1 -> GuidanceFlatEarth/3(reset_flat)
  GuidanceFlatEarth/5(flag_pos_W) -> flag_pos_W/1
  GuidanceFlatEarth/6(transition_x_target) -> transition_x_target/1
  GuidanceFlatEarth/7(Vk_desired_retraction) -> Vk_desired_retraction/1
  V_ro/1 -> GuidanceFlatEarth/4(V_ro)
  Tether_length/1 -> GuidanceFlatEarth/5(Tether_length)
  GuidanceFlatEarth/8(arcP) -> arcP/1

== system Dyn_6DoF_v2_0_R2015B/AirborneSystem/FlightControlSystem/PathFollowingController_SS_3/FlightOnSphere (Traction) ==
  reset : Inport
  phi0_update : Inport  Port=2
  FlightMode : Inport  Port=3  PortDimensions=1
  sub_flight_state : Inport  Port=4
  F_a_B_est : Inport  Port=5  PortDimensions=[3,1]
  Ft_set : Inport  Port=6
  StateEstimation_Bus : Inport  Port=7
  flag_pos_y_W : Inport  Port=8
  Compare To Constant1 : simulink/Logic and Bit Operations/Compare To Constant  Commented=on  relop===  const=5  OutDataTypeStr=boolean
  Compare To Constant2 : simulink/Logic and Bit Operations/Compare To Constant  Commented=on  relop===  const=1  OutDataTypeStr=boolean
  Constant : Constant  Value=Lbooth.init_sol
  FlightPathLoopTraction : Subsystem
  Logical Operator : Logic  Commented=on  Operator=OR  AllPortsSameDT=off  OutDataTypeStr=boolean
  Navigator : Subsystem
  Pcontroller_ChiGamma_Traction : Subsystem
  Sample and Hold : dspsigops/Sample and Hold  Commented=on  trig=Rising edge  initCond=0  latchinput=off
  Select_init_sol_for_pathfollowing : Stateflow chart  TreatAsAtomicUnit=on
  Sum : Sum  Inputs=|++
  Sum1 : Sum  Inputs=|++
  course_pathangle_error : Outport
  crosstrack_error : Outport  Port=2
  mu_a_cmd : Outport  Port=3  PortDimensions=1
  alpha_a_cmd : Outport  Port=4  PortDimensions=1
  s : Outport  Port=5
  wires:
  FlightPathLoopTraction/1(mu_a_c_traction) -> mu_a_cmd/1
  Navigator/5(course_pathangle_error) -> Pcontroller_ChiGamma_Traction/1(course_pathangle_error), course_pathangle_error/1
  Navigator/3(crosstrack_error) -> crosstrack_error/1
  FlightPathLoopTraction/2(alpha_rq) -> alpha_a_cmd/1
  F_a_B_est/1 -> FlightPathLoopTraction/2(F_a_B_est)
  Ft_set/1 -> FlightPathLoopTraction/1(Ft_set)
  StateEstimation_Bus/1 -> FlightPathLoopTraction/3(StateEstimation_Bus), Navigator/4(StateEstimation_Bus)
  Navigator/4(s) -> s/1
  phi0_update/1 -> Navigator/1(phi0_update)
  reset/1 -> Navigator/Enable, FlightPathLoopTraction/Enable
  Navigator/1(chi_k_dot) -> Sum/1
  Navigator/2(gamma_k_dot) -> Sum1/1
  Select_init_sol_for_pathfollowing/1(sol_init) -> Navigator/5(init_value)
  Constant/1 -> Select_init_sol_for_pathfollowing/1(x)
  Sum1/1 -> FlightPathLoopTraction/5(nu_gamma)
  Sum/1 -> FlightPathLoopTraction/4(nu_chi)
  FlightMode/1 -> Navigator/3(flight_mode), Sample and Hold/1, Compare To Constant2/1, Compare To Constant1/1, Select_init_sol_for_pathfollowing/2(fm)
  flag_pos_y_W/1 -> Select_init_sol_for_pathfollowing/3(flag_pos_y_W)
  Pcontroller_ChiGamma_Traction/1(Chi_cntr) -> Sum/2
  Pcontroller_ChiGamma_Traction/2(Gamma_cntr) -> Sum1/2
  Compare To Constant2/1 -> Logical Operator/1
  Compare To Constant1/1 -> Logical Operator/2
  Logical Operator/1 -> Sample and Hold/Trigger
  Sample and Hold/1 -> Navigator/6(fm_mem)
  sub_flight_state/1 -> Navigator/2(sub_flight_state)

== system Dyn_6DoF_v2_0_R2015B/AirborneSystem/ForcesAndTorques/Subsystem Reference_SS_4/Aileron1 ==
  In : Inport
  Constant : Constant  Value=Bias
  Constant2 : Constant
  Discrete-Time Integrator : DiscreteIntegrator  InitialConditionSource=external  InitialConditionSetting=State (most efficient)  SampleTime=-1  LimitOutput=on  UpperSaturationLimit=POS_hi  LowerSaturationLimit=POS_lo  ICPrevOutput=DiscIntNeverNeededParam  ICPrevScaledInput=DiscIntNeverNeededParam
  Gain : Gain  Gain=2*pi*freq  SaturateOnIntegerOverflow=on  OutDataTypeStr=Inherit: Same as input  ParamDataTypeStr=Inherit: Same as input
  Product : Product
  Rate Limiter : Saturate  UpperLimit=RL  LowerLimit=-RL
  Sum : Sum  Inputs=-+|  SaturateOnIntegerOverflow=on  InputSameDT=on  OutDataTypeStr=Inherit: Same as first input
  Sum1 : Sum  Inputs=++|  SaturateOnIntegerOverflow=on  InputSameDT=on  OutDataTypeStr=Inherit: Same as first input
  Out : Outport  PortDimensions=1
  wires:
  Constant2/1 -> Product/1
  Constant/1 -> Sum1/1
  Gain/1 -> Product/2  "Ydot"
  Sum/1 -> Gain/1  "Error"
  Discrete-Time Integrator/1 -> Sum/1, Out/1  "Y"
  Rate Limiter/1 -> Discrete-Time Integrator/1  "Ydot_lim"
  In/1 -> Sum1/2
  Sum1/1 -> Sum/2, Discrete-Time Integrator/2
  Product/1 -> Rate Limiter/1

== system Dyn_6DoF_v2_0_R2015B/AirborneSystem/ForcesAndTorques/Subsystem Reference_SS_4/Elevator ==
  In : Inport
  Constant : Constant  Value=Bias
  Discrete-Time Integrator : DiscreteIntegrator  InitialConditionSource=external  InitialConditionSetting=State (most efficient)  SampleTime=-1  LimitOutput=on  UpperSaturationLimit=POS_hi  LowerSaturationLimit=POS_lo  ICPrevOutput=DiscIntNeverNeededParam  ICPrevScaledInput=DiscIntNeverNeededParam
  Gain : Gain  Gain=2*pi*freq  SaturateOnIntegerOverflow=on  OutDataTypeStr=Inherit: Same as input  ParamDataTypeStr=Inherit: Same as input
  Rate Limiter : Saturate  UpperLimit=RL  LowerLimit=-RL
  Scope : Scope  NumInputPorts=2
  Sum : Sum  Inputs=-+|  SaturateOnIntegerOverflow=on  InputSameDT=on  OutDataTypeStr=Inherit: Same as first input
  Sum1 : Sum  Inputs=++|  SaturateOnIntegerOverflow=on  InputSameDT=on  OutDataTypeStr=Inherit: Same as first input
  Out : Outport  PortDimensions=1
  wires:
  Sum1/1 -> Discrete-Time Integrator/2, Sum/2
  In/1 -> Sum1/2
  Rate Limiter/1 -> Scope/2, Discrete-Time Integrator/1  "Ydot_lim"
  Discrete-Time Integrator/1 -> Out/1, Sum/1  "Y"
  Sum/1 -> Gain/1  "Error"
  Gain/1 -> Scope/1, Rate Limiter/1  "Ydot"
  Constant/1 -> Sum1/1

== system Dyn_6DoF_v2_0_R2015B/AirborneSystem/ForcesAndTorques/Subsystem Reference_SS_4/Rudder1 ==
  In : Inport
  Constant : Constant  Value=Bias
  Discrete-Time Integrator : DiscreteIntegrator  InitialConditionSource=external  InitialConditionSetting=State (most efficient)  SampleTime=-1  LimitOutput=on  UpperSaturationLimit=POS_hi  LowerSaturationLimit=POS_lo  ICPrevOutput=DiscIntNeverNeededParam  ICPrevScaledInput=DiscIntNeverNeededParam
  Gain : Gain  Gain=2*pi*freq  SaturateOnIntegerOverflow=on  OutDataTypeStr=Inherit: Same as input  ParamDataTypeStr=Inherit: Same as input
  Rate Limiter : Saturate  UpperLimit=RL  LowerLimit=-RL
  Sum : Sum  Inputs=-+|  SaturateOnIntegerOverflow=on  InputSameDT=on  OutDataTypeStr=Inherit: Same as first input
  Sum1 : Sum  Inputs=++|  SaturateOnIntegerOverflow=on  InputSameDT=on  OutDataTypeStr=Inherit: Same as first input
  Out : Outport  PortDimensions=1
  wires:
  Constant/1 -> Sum1/1
  Sum1/1 -> Discrete-Time Integrator/2, Sum/2
  In/1 -> Sum1/2
  Rate Limiter/1 -> Discrete-Time Integrator/1  "Ydot_lim"
  Discrete-Time Integrator/1 -> Out/1, Sum/1  "Y"
  Sum/1 -> Gain/1  "Error"
  Gain/1 -> Rate Limiter/1  "Ydot"

== system Dyn_6DoF_v2_0_R2015B/AirborneSystem/ForcesAndTorques/aerodynamic forces FSI/Elevator Aero ==
  In : Inport
  Elevator_aero : MATLAB Function  TreatAsAtomicUnit=on
  Out : Outport
  wires:
  Elevator_aero/1(out) -> Out/1
  In/1 -> Elevator_aero/1(input)

== system Dyn_6DoF_v2_0_R2015B/AirborneSystem/ForcesAndTorques/aerodynamic forces FSI/Rudder Aero ==
  In : Inport
  Rudder_aero : MATLAB Function  TreatAsAtomicUnit=on
  Out : Outport
  wires:
  Rudder_aero/1(out) -> Out/1
  In/1 -> Rudder_aero/1(input)

== system Dyn_6DoF_v2_0_R2015B/AirborneSystem/ForcesAndTorques/aerodynamic forces FSI/Subsystem ==
  alpha : Inport
  beta : Inport  Port=2
  velocity : Inport  Port=3
  Omega : Inport  Port=4
  Atan2 : Trigonometry  Operator=atan2
  Constant : Constant  Value=(DE2019.x_el+DE2019.c_el*0.25)
  Cos : Trigonometry  Operator=cos
  Cos1 : Trigonometry  Operator=cos
  Product : Product  Inputs=3
  Product1 : Product  Commented=on
  Product2 : Product  Commented=on  Inputs=3
  Product3 : Product
  Selector : Selector  InputPortWidth=3  IndexOptions=Index vector (dialog)  Indices=1  OutputSizes=1
  Sin : Trigonometry  Commented=on
  Sin1 : Trigonometry  Commented=on
  Terminator : Terminator  Commented=on
  Terminator1 : Terminator  Commented=on
  alpha_damp : Outport
  wires:
  alpha/1 -> Sin/1, Cos/1
  beta/1 -> Sin1/1, Cos1/1
  Product/1 -> Atan2/2
  Product1/1 -> Terminator/1
  Product2/1 -> Terminator1/1
  velocity/1 -> Product1/1, Product2/1, Product/1
  Cos/1 -> Product/2
  Cos1/1 -> Product2/3, Product/3
  Sin1/1 -> Product1/2
  Sin/1 -> Product2/2
  Constant/1 -> Product3/1
  Omega/1 -> Selector/1
  Selector/1 -> Product3/2
  Product3/1 -> Atan2/1
  Atan2/1 -> alpha_damp/1

== system Dyn_6DoF_v2_0_R2015B/AirborneSystem/ForcesAndTorques/aerodynamic forces FSI/Subsystem2 ==
  alpha : Inport
  beta : Inport  Port=2
  velocity : Inport  Port=3
  Omega : Inport  Port=4
  Atan2 : Trigonometry  Operator=atan2
  Constant : Constant  Value=(DE2019.x_el+DE2019.c_el*0.25)
  Cos : Trigonometry  Operator=cos
  Cos1 : Trigonometry  Operator=cos
  Gain : Gain  Gain=-1
  Product : Product  Inputs=3
  Product1 : Product  Commented=on
  Product2 : Product  Commented=on  Inputs=3
  Product3 : Product
  Selector : Selector  InputPortWidth=3  IndexOptions=Index vector (dialog)  Indices=3  OutputSizes=1
  Sin : Trigonometry  Commented=on
  Sin1 : Trigonometry  Commented=on
  beta_damp : Outport
  wires:
  Atan2/1 -> Gain/1
  Gain/1 -> beta_damp/1
  Product3/1 -> Atan2/1
  Sin1/1 -> Product1/2
  alpha/1 -> Sin/1, Cos/1
  Cos/1 -> Product/2
  Omega/1 -> Selector/1
  Sin/1 -> Product2/2
  Product1/1 -> ?
  Constant/1 -> Product3/1
  velocity/1 -> Product1/1, Product2/1, Product/1
  Product2/1 -> ?
  beta/1 -> Sin1/1, Cos1/1
  Product/1 -> Atan2/2
  Cos1/1 -> Product2/3, Product/3
  Selector/1 -> Product3/2

== system Dyn_6DoF_v2_0_R2015B/AirborneSystem/ForcesAndTorques/aerodynamic forces FSI/Wing Aero ==
  Wing_In : Inport
  time : Inport  Port=2
  Constant : Constant
  Constant1 : Constant  Value=0
  If : If  IfExpression=u1 >= 1
  If Action Subsystem : Subsystem  TreatAsAtomicUnit=on
  If Action Subsystem1 : Subsystem  TreatAsAtomicUnit=on
  Merge : Merge
  Switch : Switch  Threshold=simInit.FSI_switchtime
  Wing_Out : Outport
  wires:
  If/1 -> If Action Subsystem/Action
  If/2 -> If Action Subsystem1/Action
  If Action Subsystem1/1(Simple_out) -> Merge/2
  If Action Subsystem/1(FSI_out) -> Merge/1
  Merge/1 -> Wing_Out/1
  time/1 -> Switch/2, If Action Subsystem/2(simTime)
  Constant/1 -> Switch/1
  Constant1/1 -> Switch/3
  Switch/1 -> If/1
  Wing_In/1 -> If Action Subsystem1/1(Simple_in), If Action Subsystem/1(FSI_in)

== system Dyn_6DoF_v2_0_R2015B/Environment_SS_5/Windshear/Wind Shear Model/wind_field_calc ==
  Altitude : Inport
  Base_windspeed : Inport  Port=2
  1-D Lookup Table : Lookup_n-D  NumberOfTableDimensions=1  BreakpointsForDimension1=ENVMT.wind_height  Table=ENVMT.wind_data  InternalRulePriority=Speed  RndMeth=Simplest  InputSameDT=on
  3ft-->inf : Saturate  Commented=on  UpperLimit=inf  LowerLimit=3
  Length Conversion : Subsystem  Commented=on
  Manual Switch : ManualSwitch  CurrentSetting=0
  Product : Product  Commented=on  Inputs=*/  SaturateOnIntegerOverflow=on  InputSameDT=on  OutDataTypeStr=Inherit: Same as first input
  Product1 : Product  Commented=on  SaturateOnIntegerOverflow=on  InputSameDT=on  OutDataTypeStr=Inherit: Same as first input
  Product2 : Product  SaturateOnIntegerOverflow=on  InputSameDT=on  OutDataTypeStr=Inherit: Same as first input
  Reshape : Reshape  OutputDimensionality=Column vector (2-D)
  Saturation : Saturate  UpperLimit=ENVMT.height_max  LowerLimit=ENVMT.wind_height(1)
  h/z0 : Gain  Commented=on  Gain=1/0.15  SaturateOnIntegerOverflow=on  OutDataTypeStr=Inherit: Same as input  ParamDataTypeStr=Inherit: Same as input
  ln(h/z0) : Math  Commented=on  Operator=log  SaturateOnIntegerOverflow=on
  ln(ref_height/z0) : Math  Commented=on  Operator=log  SaturateOnIntegerOverflow=on
  ref_height/z0 [ft] : Constant  Commented=on  Value=20/0.15  OutDataTypeStr=Inherit: Inherit via back propagation
  Windspeed_altitude : Outport
  wires:
  Altitude/1 -> Saturation/1, Length Conversion/1(in)
  ref_height/z0 [ft]/1 -> ln(ref_height/z0)/1
  h/z0/1 -> ln(h/z0)/1
  Product/1 -> Product1/1
  Manual Switch/1 -> Reshape/1
  Saturation/1 -> 1-D Lookup Table/1  "ijmuiden"
  Base_windspeed/1 -> Product2/2, Product1/2
  Product1/1 -> Manual Switch/1  "log-law"
  Length Conversion/1(out) -> 3ft-->inf/1
  ln(h/z0)/1 -> Product/1
  Reshape/1 -> Windspeed_altitude/1
  1-D Lookup Table/1 -> Product2/1
  ln(ref_height/z0)/1 -> Product/2
  Product2/1 -> Manual Switch/2  "referencce location"
  3ft-->inf/1 -> h/z0/1

== system Dyn_6DoF_v2_0_R2015B/AirborneSystem/FlightControlSystem/AirspeedController_SS_1/Airspeed_Brake/Subsystem ==
  V_cmd : Inport
  v_h : Inport  Port=2
  Initial : Inport  Port=3
  Discrete-Time Integrator1 : DiscreteIntegrator  InitialConditionSource=external  InitialCondition=norm(simInit.vel_B_init)  InitialConditionSetting=State (most efficient)  SampleTime=-1  LimitOutput=on  UpperSaturationLimit=120  LowerSaturationLimit=0  ICPrevOutput=DiscIntNeverNeededParam  ICPrevScaledInput=DiscIntNeverNeededParam
  Gain2 : Gain  Gain=params.w0SpeedControl  Multiplication=Matrix(K*u)
  Sum1 : Sum  Inputs=|+-
  Sum2 : Sum  Inputs=|+-
  V_k_ref : Outport
  wires:
  Gain2/1 -> Sum1/1
  v_h/1 -> Sum1/2
  Sum1/1 -> Discrete-Time Integrator1/1
  V_cmd/1 -> Sum2/1
  Sum2/1 -> Gain2/1
  Discrete-Time Integrator1/1 -> Sum2/2, V_k_ref/1
  Initial/1 -> Discrete-Time Integrator1/2

== system Dyn_6DoF_v2_0_R2015B/AirborneSystem/FlightControlSystem/AirspeedController_SS_1/Airspeed_Control/Subsystem ==
  V_cmd : Inport
  v_h : Inport  Port=2
  Discrete-Time Integrator1 : DiscreteIntegrator  InitialCondition=norm(simInit.vel_B_init)  InitialConditionSetting=State (most efficient)  SampleTime=-1  LimitOutput=on  UpperSaturationLimit=120  LowerSaturationLimit=0  ICPrevOutput=DiscIntNeverNeededParam  ICPrevScaledInput=DiscIntNeverNeededParam
  Gain2 : Gain  Gain=params.w0SpeedControl  Multiplication=Matrix(K*u)
  Sum1 : Sum  Inputs=|+-
  Sum2 : Sum  Inputs=|+-
  V_k_ref_dot : Outport
  V_k_ref : Outport  Port=2
  wires:
  Gain2/1 -> Sum1/1, V_k_ref_dot/1
  v_h/1 -> Sum1/2
  Sum1/1 -> Discrete-Time Integrator1/1
  V_cmd/1 -> Sum2/1
  Sum2/1 -> Gain2/1
  Discrete-Time Integrator1/1 -> V_k_ref/1, Sum2/2

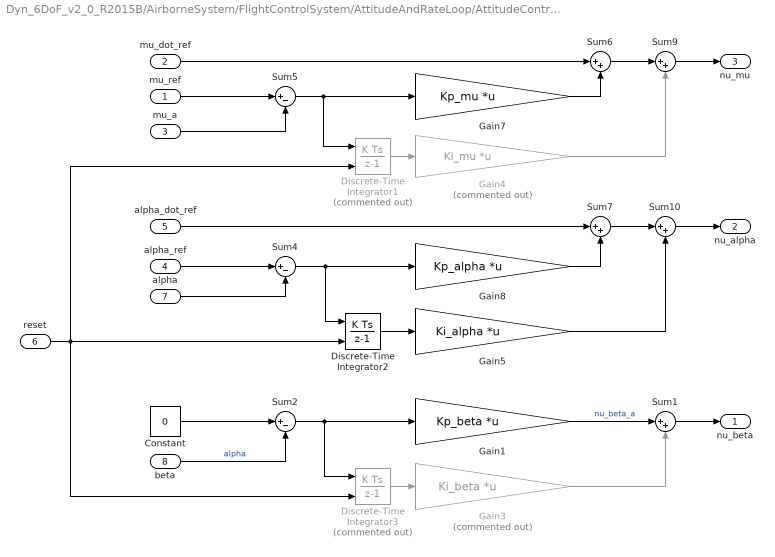
== system Dyn_6DoF_v2_0_R2015B/AirborneSystem/FlightControlSystem/AttitudeAndRateLoop/AttitudeController/PI-controller ==
  mu_ref : Inport
  mu_dot_ref : Inport  Port=2
  mu_a : Inport  Port=3
  alpha_ref : Inport  Port=4
  alpha_dot_ref : Inport  Port=5
  reset : Inport  Port=6
  alpha : Inport  Port=7
  beta : Inport  Port=8
  Constant : Constant  Value=0
  Discrete-Time Integrator1 : DiscreteIntegrator  Commented=on  ExternalReset=rising  InitialConditionSetting=State (most efficient)  SampleTime=-1  ICPrevOutput=DiscIntNeverNeededParam  ICPrevScaledInput=DiscIntNeverNeededParam
  Discrete-Time Integrator2 : DiscreteIntegrator  ExternalReset=either  InitialConditionSetting=State (most efficient)  SampleTime=-1  ICPrevOutput=DiscIntNeverNeededParam  ICPrevScaledInput=DiscIntNeverNeededParam
  Discrete-Time Integrator3 : DiscreteIntegrator  Commented=on  ExternalReset=rising  InitialConditionSetting=State (most efficient)  SampleTime=-1  ICPrevOutput=DiscIntNeverNeededParam  ICPrevScaledInput=DiscIntNeverNeededParam
  Gain1 : Gain  Gain=Kp_beta  Multiplication=Matrix(K*u)
  Gain3 : Gain  Commented=on  Gain=Ki_beta  Multiplication=Matrix(K*u)
  Gain4 : Gain  Commented=on  Gain=Ki_mu  Multiplication=Matrix(K*u)
  Gain5 : Gain  Gain=Ki_alpha  Multiplication=Matrix(K*u)
  Gain7 : Gain  Gain=Kp_mu  Multiplication=Matrix(K*u)
  Gain8 : Gain  Gain=Kp_alpha  Multiplication=Matrix(K*u)
  Sum{1,6..7,9..10} (5 alike) : Sum  Inputs=|++
  Sum2 : Sum  Inputs=|+-
  Sum4 : Sum  Inputs=|+-
  Sum5 : Sum  Inputs=|+-
  nu_beta : Outport
  nu_alpha : Outport  Port=2
  nu_mu : Outport  Port=3
  wires:
  Gain8/1 -> Sum7/2
  Gain5/1 -> Sum10/2
  Gain4/1 -> Sum9/2
  Sum7/1 -> Sum10/1
  Sum6/1 -> Sum9/1
  Gain7/1 -> Sum6/2
  Discrete-Time Integrator1/1 -> Gain4/1
  Sum4/1 -> Discrete-Time Integrator2/1, Gain8/1
  Sum5/1 -> Discrete-Time Integrator1/1, Gain7/1
  alpha/1 -> Sum4/2
  mu_a/1 -> Sum5/2
  alpha_ref/1 -> Sum4/1
  mu_ref/1 -> Sum5/1
  alpha_dot_ref/1 -> Sum7/1
  mu_dot_ref/1 -> Sum6/1
  reset/1 -> Discrete-Time Integrator2/2, Discrete-Time Integrator3/2, Discrete-Time Integrator1/2
  Constant/1 -> Sum2/1
  Sum2/1 -> Discrete-Time Integrator3/1, Gain1/1
  Gain1/1 -> Sum1/1  "nu_beta_a"
  beta/1 -> Sum2/2  "alpha"
  Gain3/1 -> Sum1/2
  Discrete-Time Integrator3/1 -> Gain3/1
  Sum1/1 -> nu_beta/1
  Sum10/1 -> nu_alpha/1
  Sum9/1 -> nu_mu/1
  Discrete-Time Integrator2/1 -> Gain5/1
